simulink library "DYN_ATT"  (Simulink 8.8)
settings: Solver=ode45  StartTime=0.0  StopTime=10.0  RelTol=1e-3  EnableMultiTasking=on
libraries: LIB_DYN x1
settings Model: Creator=alger  LastModifiedBy=alger

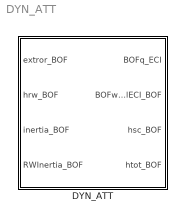
== system DYN_ATT ==
  DYN_ATT : Subsystem

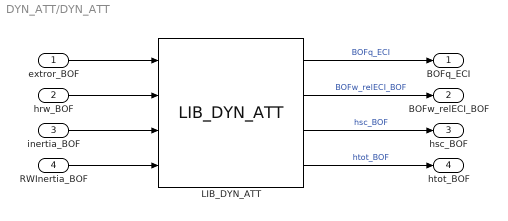
== system DYN_ATT/DYN_ATT ==
  extror_BOF : Inport
  hrw_BOF : Inport  Port=2
  inertia_BOF : Inport  Port=3
  RWInertia_BOF : Inport  Port=4
  LIB_DYN_ATT : LIB_DYN/LIB_DYN_ATT  BOFq_CEL_ini=DYN_ATT_par.BOFq_ECI_ini  h_BOF_ini=DYN_ATT_par.h_BOF_ini  zero_tol=CONSTANTS_par.zero_tol
  BOFq_ECI : Outport
  BOFw_relECI_BOF : Outport  Port=2
  hsc_BOF : Outport  Port=3
  htot_BOF : Outport  Port=4
  wires:
  LIB_DYN_ATT/3 -> hsc_BOF/1  "hsc_BOF"
  LIB_DYN_ATT/1 -> BOFq_ECI/1  "BOFq_ECI"
  LIB_DYN_ATT/4 -> htot_BOF/1  "htot_BOF"
  inertia_BOF/1 -> LIB_DYN_ATT/3
  extror_BOF/1 -> LIB_DYN_ATT/1
  hrw_BOF/1 -> LIB_DYN_ATT/2
  RWInertia_BOF/1 -> LIB_DYN_ATT/4
  LIB_DYN_ATT/2 -> BOFw_relECI_BOF/1  "BOFw_relECI_BOF"
